simulink model "wheel_leg"  (R2024b)
settings: Solver=FixedStepAuto  StartTime=0.0  StopTime=10  FixedStep=0.001  RelTol=1e-3  AbsTol=1e-3  EnableMultiTasking=on
model workspace: external: MATLAB File UseBodyVel.m (data not in the file)
values from neighbouring files (symbols this model uses):
  g = 9.81    [LQR_calc.m]    (also in UseBodyVel.m)
  joint_distance = 0.11    [LQR_calc.m]    (also in UseBodyVel.m)
  l = -0.014    [LQR_calc.m]    (also in UseBodyVel.m)
  l_active_leg = 0.14    [LQR_calc.m]    (also in UseBodyVel.m)
  l_slave_leg = 0.24    [LQR_calc.m]    (also in UseBodyVel.m)
  M = 12    [LQR_calc.m]    (also in UseBodyVel.m)
  m_active_leg = 0.174    [LQR_calc.m]    (also in UseBodyVel.m)
  m_slave_leg = 0.180    (= 0.18)    [LQR_calc.m]    (also in UseBodyVel.m)
  mw = 0.58    [LQR_calc.m]    (also in UseBodyVel.m)
  N = mp*(x_ddot+L*theta_ddot*cos(theta)-L*theta_dot^2*sin(theta))+N_M    [UseBodyVel.m]
  X = [theta,theta_dot,x,x_dot,phi,phi_dot].'    [UseBodyVel.m]
undefined symbols (not defined in the file or in its folder): Y, Z
libraries: sm_lib x65, nesl_utility x25, dspfdesign x3
(part 1 of 3)
settings Model: Creator=kai  LastModifiedBy=kai
settings SolverCC: AutoScaleAbsTol=off  AlgebraicLoopSolver=TrustRegion  MaxZcPerStep=1
settings DataIOCC: LimitDataPoints=on  MaxDataPoints=10000
settings OptimizationCC: ReuseModelBlockBuffer=off  LifeSpan=inf
settings DebuggingCC: UnconnectedInputMsg=warning  UnconnectedOutputMsg=warning  UnconnectedLineMsg=warning  AllowSymbolicDim=off  SFUnexpectedBacktrackingDiag=warning  SFNoUnconditionalDefaultTransitionDiag=warning  SFExecutionAtInitializationDiag=none  ArithmeticOperatorsInVariantConditions=warning
settings ModelReferenceCC: EnableRefExpFcnMdlSchedulingChecks=on
settings SFSimCC: SimUseLocalCustomCode=off  CustomCodeUndefinedFunction=UseInterfaceOnly
settings RTWCC: RTWUseLocalCustomCode=off  GPUComputeCapability=3.5  DLArmComputeVersion=19.05
settings CodeAppCC: StateflowObjectComments=on
settings GRTTargetCC: TargetLangStandard=C89/C90 (ANSI)
settings ConfigComp: CovMetricSettings=dw  CovSaveCumulativeToWorkspaceVar=on  CovSaveSingleToWorkspaceVar=on  CovExternalEMLEnable=off  CovSFcnEnable=off
settings SimscapeCC: SimscapeLogType=all  SimscapeLogSimulationStatistics=on  SimscapeLogDataHistory=10000

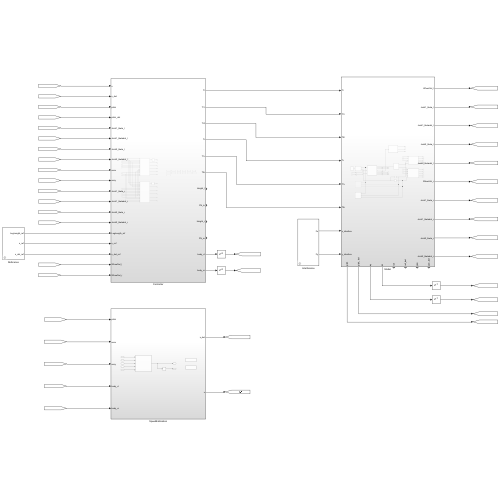
[thumbnail: Simulink's stored preview of the top-level diagram]
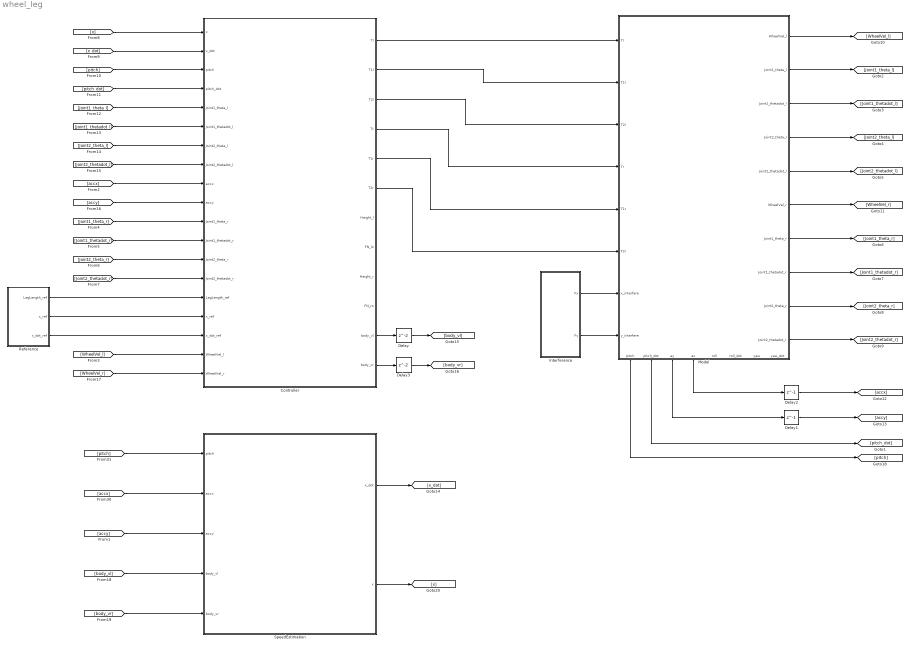
== system wheel_leg ==
  Controller : Subsystem
  Delay : Delay
  Delay1 : Delay  DelayLength=1
  Delay2 : Delay  DelayLength=1
  Delay3 : Delay
  Interference : Subsystem  mask{Fx=0, Fy=0}
      mask prompts: Fx "Fx（N）"; Fy "Fy（N）"
      mask DialogControl ParameterGroupVar Prompt: 参数
  Model : Subsystem
      settings: PortSchema="{\"entries\":[{\"content\":{\"sides\":[{\"content\":{\"connectorIds\":[\"In1\",\"In2\",\"In3\",\"In4\",\"In5\",\"In6\",\"In7\",\"In8\"]},\"type\":\"ConnectorPlacement.EquallySpacedRectSide\",\"uuid\":\"a2ef8d1c-db40-41d8-a076-97a3cc9cbcfc\"},{\"content\":{\"connectorIds\":[\"Out1\",\"Out2\",\"Out3\",\"Out4\",\"Out5\",\"Out6\",\"Out7\",\"Out8\",\"Out9\",\"Out10\"],\"side\":\"RIGHT\"},\"type\":\"ConnectorPlacement.EquallySpacedRectSide\",\"uuid\":\"78dabc19-8860-4beb-a8ed-91b17f10298d\"},{\"content\":{\"side\":\"TOP\"},\"type\":\"ConnectorPlacement.EquallySpacedRectSide\",\"uuid\":\"c54bf74f-6f46-45cf-a87a-01175e203e11\"},{\"content\":{\"connectorIds\":[\"Out11\",\"Out12\",\"Out13\",\"Out14\",\"Out15\",\"Out16\",\"Out17\",\"Out18\"],\"side\":\"BOTTOM\"},\"type\":\"ConnectorPlacement.EquallySpacedRectSide\",\"uuid\":\"b0255ca1-76d0-4c58-9ab3-44ef179b6807\"}]},\"type\":\"ConnectorPlacement.EquallySpacedConnector\",\"uuid\":\"6cb8f578-1c5f-4fff-8912-748653416d88\"}],\"packageUris\":[\"http://schema.mathworks.com/mf0/Connector/R2020b\"],\"version\":\"1.0\"}"
  Reference : Subsystem  mask{LegLength_expe=0.3, vel_expe=3, conti_time=7}
      mask prompts: LegLength_expe "腿长期望(m)"; vel_expe "速度期望(m/s)"; conti_time "速度持续时间(s)"
      mask DialogControl ParameterGroupVar Prompt: 参数
  SpeedEstimation : Subsystem
  wires:
  Model/2(Joint1_theta_l) -> [Joint1_theta_l]
  Model/3(Joint1_thetadot_l) -> [Joint1_thetadot_l]
  Model/4(Joint2_theta_l) -> [Joint2_theta_l]
  Model/5(Joint2_thetadot_l) -> [Joint2_thetadot_l]
  Model/7(Joint1_theta_r) -> [Joint1_theta_r]
  Model/8(Joint1_thetadot_r) -> [Joint1_thetadot_r]
  Model/9(Joint2_theta_r) -> [Joint2_theta_r]
  Model/10(Joint2_thetadot_r) -> [Joint2_thetadot_r]
  Model/1(WheelVel_l) -> [WheelVel_l]
  Model/6(WheelVel_r) -> [WheelVel_r]
  Model/11(pitch) -> [pitch]
  Model/12(pitch_dot) -> [pitch_dot]
  Model/13(ay) -> Delay1/1
  Delay1/1 -> [accy]
  Model/14(ax) -> Delay2/1
  Delay2/1 -> [accx]
  [pitch] -> SpeedEstimation/1(pitch)
  [accx] -> SpeedEstimation/2(accx)
  [x] -> Controller/1(x)
  [x_dot] -> Controller/2(x_dot)
  [pitch] -> Controller/3(pitch)
  [pitch_dot] -> Controller/4(pitch_dot)
  [Joint1_theta_l] -> Controller/5(Joint1_theta_l)
  [Joint1_thetadot_l] -> Controller/6(Joint1_thetadot_l)
  [Joint2_theta_l] -> Controller/7(Joint2_theta_l)
  [Joint2_thetadot_l] -> Controller/8(Joint2_thetadot_l)
  [accy] -> Controller/10(accy)
  [Joint1_theta_r] -> Controller/11(Joint1_theta_r)
  [Joint1_thetadot_r] -> Controller/12(Joint1_thetadot_r)
  [Joint2_theta_r] -> Controller/13(Joint2_theta_r)
  [Joint2_thetadot_r] -> Controller/14(Joint2_thetadot_r)
  Reference/1(LegLength_ref) -> Controller/15(LegLength_ref)
  Reference/2(x_ref) -> Controller/16(x_ref)
  Reference/3(x_dot_ref) -> Controller/17(x_dot_ref)
  Controller/1(Tl) -> Model/1(Tl)
  Controller/2(T1l) -> Model/2(T1l)
  Controller/3(T2l) -> Model/3(T2l)
  Controller/4(Tr) -> Model/4(Tr)
  Controller/5(T1r) -> Model/5(T1r)
  Controller/6(T2r) -> Model/6(T2r)
  [accx] -> Controller/9(accx)
  [accy] -> SpeedEstimation/3(accy)
  SpeedEstimation/1(x_dot) -> [x_dot]
  SpeedEstimation/2(x) -> [x]
  [WheelVel_l] -> Controller/18(WheelVel_l)
  [WheelVel_r] -> Controller/19(WheelVel_r)
  [body_vl] -> SpeedEstimation/4(body_vl)
  [body_vr] -> SpeedEstimation/5(body_vr)
  Controller/11(body_vl) -> Delay/1
  Delay/1 -> [body_vl]
  Controller/12(body_vr) -> Delay3/1
  Delay3/1 -> [body_vr]
  Interference/2(Fy) -> Model/8(y_interfere)
  Interference/1(Fx) -> Model/7(x_interfere)

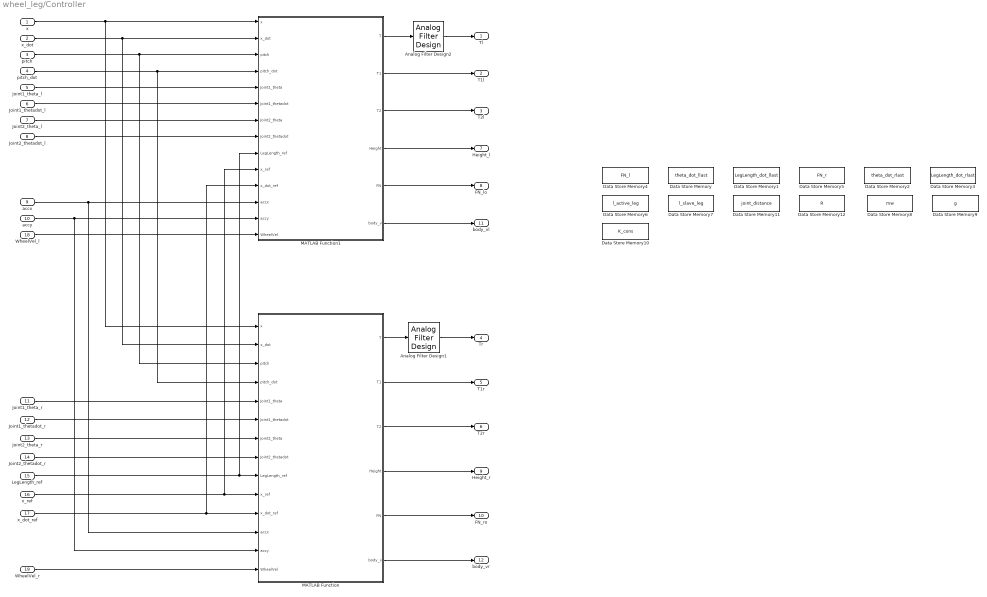
== system wheel_leg/Controller ==
  x : Inport
  x_dot : Inport  Port=2
  pitch : Inport  Port=3
  pitch_dot : Inport  Port=4
  Joint1_theta_l : Inport  Port=5
  Joint1_thetadot_l : Inport  Port=6
  Joint2_theta_l : Inport  Port=7
  Joint2_thetadot_l : Inport  Port=8
  accx : Inport  Port=9
  accy : Inport  Port=10
  Joint1_theta_r : Inport  Port=11
  Joint1_thetadot_r : Inport  Port=12
  Joint2_theta_r : Inport  Port=13
  Joint2_thetadot_r : Inport  Port=14
  LegLength_ref : Inport  Port=15
  x_ref : Inport  Port=16
  x_dot_ref : Inport  Port=17
  WheelVel_l : Inport  Port=18
  WheelVel_r : Inport  Port=19
  Analog Filter Design1 : dspfdesign/Analog Filter Design  method=Butterworth  filttype=Lowpass  N=1  Wlo=100  Whi=80  Rp=2  Rs=40
  Analog Filter Design2 : dspfdesign/Analog Filter Design  method=Butterworth  filttype=Lowpass  N=1  Wlo=100  Whi=80  Rp=2  Rs=40
  Data Store Memory : DataStoreMemory  DataStoreName=theta_dot_llast  WriteAfterWriteMsg=warning  ShowAdditionalParam=off  OutDataTypeStr=double
  Data Store Memory1 : DataStoreMemory  DataStoreName=LegLength_dot_llast  WriteAfterWriteMsg=warning  ShowAdditionalParam=off  OutDataTypeStr=double
  Data Store Memory10 : DataStoreMemory  DataStoreName=K_cons  WriteAfterWriteMsg=warning  InitialValue=K_cons  VectorParams1D=off  ShowAdditionalParam=off  OutDataTypeStr=double
  Data Store Memory11 : DataStoreMemory  DataStoreName=joint_distance  WriteAfterWriteMsg=warning  InitialValue=joint_distance  ShowAdditionalParam=off  OutDataTypeStr=double
  Data Store Memory12 : DataStoreMemory  DataStoreName=R  WriteAfterWriteMsg=warning  InitialValue=R  ShowAdditionalParam=off  OutDataTypeStr=double
  Data Store Memory2 : DataStoreMemory  DataStoreName=theta_dot_rlast  WriteAfterWriteMsg=warning  ShowAdditionalParam=off  OutDataTypeStr=double
  Data Store Memory3 : DataStoreMemory  DataStoreName=LegLength_dot_rlast  WriteAfterWriteMsg=warning  ShowAdditionalParam=off  OutDataTypeStr=double
  Data Store Memory4 : DataStoreMemory  DataStoreName=FN_l  WriteAfterWriteMsg=warning  InitialValue=70  ShowAdditionalParam=off  OutDataTypeStr=double
  Data Store Memory5 : DataStoreMemory  DataStoreName=FN_r  WriteAfterWriteMsg=warning  InitialValue=70  ShowAdditionalParam=off  OutDataTypeStr=double
  Data Store Memory6 : DataStoreMemory  DataStoreName=l_active_leg  WriteAfterWriteMsg=warning  InitialValue=l_active_leg  ShowAdditionalParam=off  OutDataTypeStr=double
  Data Store Memory7 : DataStoreMemory  DataStoreName=l_slave_leg  WriteAfterWriteMsg=warning  InitialValue=l_slave_leg  ShowAdditionalParam=off  OutDataTypeStr=double
  Data Store Memory8 : DataStoreMemory  DataStoreName=mw  WriteAfterWriteMsg=warning  InitialValue=mw  ShowAdditionalParam=off  OutDataTypeStr=double
  Data Store Memory9 : DataStoreMemory  DataStoreName=g  WriteAfterWriteMsg=warning  InitialValue=g  ShowAdditionalParam=off  OutDataTypeStr=double
  MATLAB Function : MATLAB Function  TreatAsAtomicUnit=on
  MATLAB Function1 : MATLAB Function  TreatAsAtomicUnit=on
  Tl : Outport
  T1l : Outport  Port=2
  T2l : Outport  Port=3
  Tr : Outport  Port=4
  T1r : Outport  Port=5
  T2r : Outport  Port=6
  Height_l : Outport  Port=7
  FN_lo : Outport  Port=8
  Height_r : Outport  Port=9
  FN_ro : Outport  Port=10
  body_vl : Outport  Port=11
  body_vr : Outport  Port=12
  wires:
  LegLength_ref/1 -> MATLAB Function/9(LegLength_ref), MATLAB Function1/9(LegLength_ref)
  MATLAB Function1/3(T2) -> T2l/1
  x_ref/1 -> MATLAB Function1/10(x_ref), MATLAB Function/10(x_ref)
  x_dot_ref/1 -> MATLAB Function1/11(x_dot_ref), MATLAB Function/11(x_dot_ref)
  MATLAB Function/1(T) -> Analog Filter Design1/1
  MATLAB Function/2(T1) -> T1r/1
  Analog Filter Design2/1 -> Tl/1
  MATLAB Function/3(T2) -> T2r/1
  Joint2_theta_r/1 -> MATLAB Function/7(Joint2_theta)
  Joint2_thetadot_r/1 -> MATLAB Function/8(Joint2_thetadot)
  MATLAB Function1/2(T1) -> T1l/1
  pitch_dot/1 -> MATLAB Function1/4(pitch_dot), MATLAB Function/4(pitch_dot)
  Joint1_thetadot_l/1 -> MATLAB Function1/6(Joint1_thetadot)
  Joint1_theta_r/1 -> MATLAB Function/5(Joint1_theta)
  MATLAB Function/5(FN) -> FN_ro/1
  x/1 -> MATLAB Function1/1(x), MATLAB Function/1(x)
  Joint1_thetadot_r/1 -> MATLAB Function/6(Joint1_thetadot)
  Joint2_theta_l/1 -> MATLAB Function1/7(Joint2_theta)
  Joint1_theta_l/1 -> MATLAB Function1/5(Joint1_theta)
  Analog Filter Design1/1 -> Tr/1
  accy/1 -> MATLAB Function/13(accy), MATLAB Function1/13(accy)
  Joint2_thetadot_l/1 -> MATLAB Function1/8(Joint2_thetadot)
  x_dot/1 -> MATLAB Function1/2(x_dot), MATLAB Function/2(x_dot)
  pitch/1 -> MATLAB Function1/3(pitch), MATLAB Function/3(pitch)
  MATLAB Function1/4(Height) -> Height_l/1
  MATLAB Function1/5(FN) -> FN_lo/1
  MATLAB Function/4(Height) -> Height_r/1
  accx/1 -> MATLAB Function/12(accx), MATLAB Function1/12(accx)
  MATLAB Function1/1(T) -> Analog Filter Design2/1
  WheelVel_l/1 -> MATLAB Function1/14(WheelVel)
  WheelVel_r/1 -> MATLAB Function/14(WheelVel)
  MATLAB Function1/6(body_v) -> body_vl/1
  MATLAB Function/6(body_v) -> body_vr/1

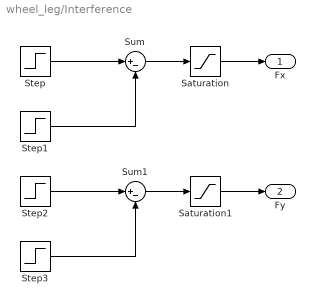
== system wheel_leg/Interference ==
  Saturation : Saturate  UpperLimit=80  LowerLimit=-80
  Saturation1 : Saturate  UpperLimit=100  LowerLimit=-100
  Step : Step  Time=0.5  After=Fx  SampleTime=0
  Step1 : Step  Time=0.6  After=Fx  SampleTime=0
  Step2 : Step  Time=0.5  After=Fy  SampleTime=0
  Step3 : Step  Time=0.6  After=Fy  SampleTime=0
  Sum : Sum  Inputs=|+-
  Sum1 : Sum  Inputs=|+-
  Fx : Outport
  Fy : Outport  Port=2
  wires:
  Step/1 -> Sum/1
  Step1/1 -> Sum/2
  Sum/1 -> Saturation/1
  Sum1/1 -> Saturation1/1
  Step3/1 -> Sum1/2
  Step2/1 -> Sum1/1
  Saturation/1 -> Fx/1
  Saturation1/1 -> Fy/1

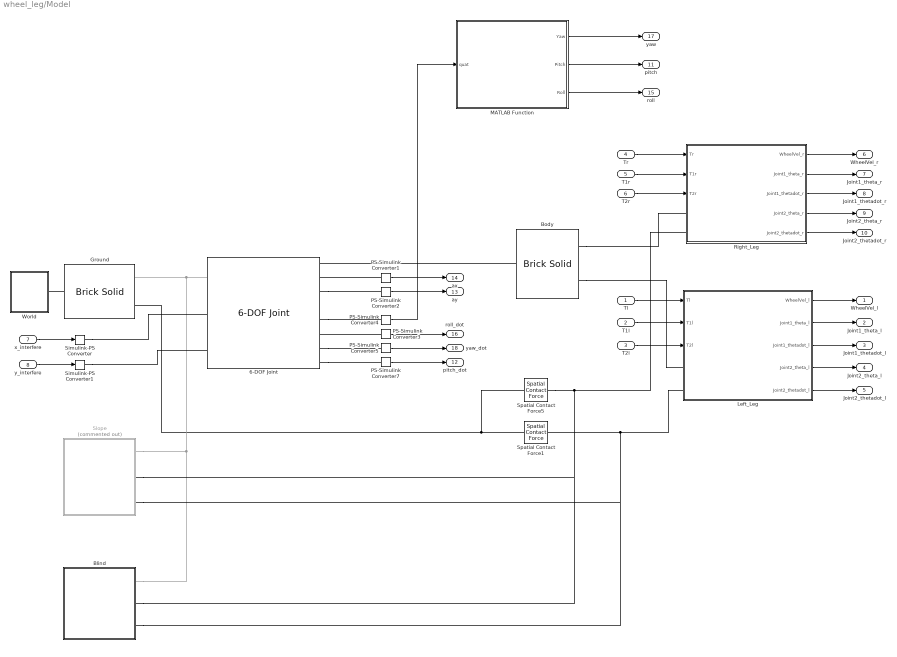
== system wheel_leg/Model ==
  Tl : Inport
  T1l : Inport  Port=2
  T2l : Inport  Port=3
  Tr : Inport  Port=4
  T1r : Inport  Port=5
  T2r : Inport  Port=6
  x_interfere : Inport  Port=7
  y_interfere : Inport  Port=8
  6-DOF Joint : sm_lib/Joints/6-DOF Joint  JointMode=Normal  CompositeWrenchDir=FollowerOnBase  CompositeWrenchFrame=BaseFrame  SenseConstraintForce=off  SenseConstraintTorque=off  SenseTotalForce=off  SenseTotalTorque=off  PxPositionTargetSpecify=off  PxPositionTargetPriority=High  PxPositionTargetValue=0  PxPositionTargetValueUnits=m  PxVelocityTargetSpecify=off  PxVelocityTargetPriority=High  PxVelocityTargetValue=0  PxVelocityTargetValueUnits=m/s  PxEquilibriumPosition=0  PxEquilibriumPositionUnits=m  PxSpringStiffness=0  PxSpringStiffnessUnits=N/m  PxDampingCoefficient=0  PxDampingCoefficientUnits=N/(m/s)  PxLowerLimitSpecify=off  PxLowerLimitBound=-1  PxLowerLimitBoundUnits=m  PxLowerLimitStiffness=1e6  PxLowerLimitStiffnessUnits=N/m  PxLowerLimitDamping=1e3  PxLowerLimitDampingUnits=N/(m/s)  PxLowerLimitTransitionRegionWidth=1e-4  PxLowerLimitTransitionRegionWidthUnits=m  PxUpperLimitSpecify=off  PxUpperLimitBound=1  PxUpperLimitBoundUnits=m  PxUpperLimitStiffness=1e6  PxUpperLimitStiffnessUnits=N/m  PxUpperLimitDamping=1e3  PxUpperLimitDampingUnits=N/(m/s)  PxUpperLimitTransitionRegionWidth=1e-4  PxUpperLimitTransitionRegionWidthUnits=m  PxTorqueActuationMode=InputTorque  PxMotionActuationMode=ComputedMotion  PxSensePosition=off  PxSenseVelocity=off  PxSenseAcceleration=on  PxSenseTorqueForce=off  PxSenseLowerLimitTorqueForce=off  PxSenseUpperLimitTorqueForce=off  PyPositionTargetSpecify=on  PyPositionTargetPriority=High  PyPositionTargetValue=0.33  PyPositionTargetValueUnits=m  PyVelocityTargetSpecify=off  PyVelocityTargetPriority=High  PyVelocityTargetValue=0  PyVelocityTargetValueUnits=m/s  PyEquilibriumPosition=0  PyEquilibriumPositionUnits=m  PySpringStiffness=0  PySpringStiffnessUnits=N/m  PyDampingCoefficient=0  PyDampingCoefficientUnits=N/(m/s)  PyLowerLimitSpecify=off  PyLowerLimitBound=-1  PyLowerLimitBoundUnits=m  PyLowerLimitStiffness=1e6  PyLowerLimitStiffnessUnits=N/m  PyLowerLimitDamping=1e3  PyLowerLimitDampingUnits=N/(m/s)  PyLowerLimitTransitionRegionWidth=1e-4  PyLowerLimitTransitionRegionWidthUnits=m  PyUpperLimitSpecify=off  PyUpperLimitBound=1  PyUpperLimitBoundUnits=m  PyUpperLimitStiffness=1e6  PyUpperLimitStiffnessUnits=N/m  PyUpperLimitDamping=1e3  PyUpperLimitDampingUnits=N/(m/s)  PyUpperLimitTransitionRegionWidth=1e-4  PyUpperLimitTransitionRegionWidthUnits=m  PyTorqueActuationMode=InputTorque  PyMotionActuationMode=ComputedMotion  PySensePosition=off  PySenseVelocity=off  PySenseAcceleration=on  PySenseTorqueForce=off  PySenseLowerLimitTorqueForce=off  PySenseUpperLimitTorqueForce=off  PzPositionTargetSpecify=off  PzPositionTargetPriority=High  PzPositionTargetValue=0  PzPositionTargetValueUnits=m  PzVelocityTargetSpecify=off  PzVelocityTargetPriority=High  PzVelocityTargetValue=0  PzVelocityTargetValueUnits=m/s  PzEquilibriumPosition=0  PzEquilibriumPositionUnits=m  PzSpringStiffness=0  PzSpringStiffnessUnits=N/m  PzDampingCoefficient=0  PzDampingCoefficientUnits=N/(m/s)  PzLowerLimitSpecify=off  PzLowerLimitBound=-1  PzLowerLimitBoundUnits=m  PzLowerLimitStiffness=1e6  PzLowerLimitStiffnessUnits=N/m  PzLowerLimitDamping=1e3  PzLowerLimitDampingUnits=N/(m/s)  PzLowerLimitTransitionRegionWidth=1e-4  PzLowerLimitTransitionRegionWidthUnits=m  PzUpperLimitSpecify=off  PzUpperLimitBound=1  PzUpperLimitBoundUnits=m  PzUpperLimitStiffness=1e6  PzUpperLimitStiffnessUnits=N/m  PzUpperLimitDamping=1e3  PzUpperLimitDampingUnits=N/(m/s)  PzUpperLimitTransitionRegionWidth=1e-4  PzUpperLimitTransitionRegionWidthUnits=m  PzTorqueActuationMode=NoTorque  PzMotionActuationMode=ComputedMotion  PzSensePosition=off  PzSenseVelocity=off  PzSenseAcceleration=on  PzSenseTorqueForce=off  PzSenseLowerLimitTorqueForce=off  PzSenseUpperLimitTorqueForce=off  SphPositionTargetSpecify=off  SphPositionTargetPriority=High  SphPositionTargetRotationMethod=None  SphPositionTargetFollAlignAxisA=+X  SphPositionTargetBaseAlignAxisA=+Y  SphPositionTargetFollAlignAxisB=+Y  SphPositionTargetBaseAlignAxisB=+Z  SphPositionTargetRotationStandardAxis=+Z  SphPositionTargetRotationAngle=0.0  SphPositionTargetRotationAngleUnits=deg  SphPositionTargetRotationArbitraryAxis=[0 0 1]  SphPositionTargetRotationSequenceAxes=FollowerAxes  SphPositionTargetRotationSequence=XYX  SphPositionTargetRotationSequenceAngles=[0 0 0]  SphPositionTargetRotationSequenceAnglesUnits=deg  SphPositionTargetRotationMatrix=[1 0 0; 0 1 0; 0 0 1]  SphPositionTargetQuaternion=[1 0 0 0]  SphVelocityTargetSpecify=off  SphVelocityTargetPriority=High  SphVelocityTargetValue=[0 0 0]  SphVelocityTargetValueUnits=deg/s  SphVelocityTargetInFollowerFrame=on  SphEqPosRotationMethod=None  SphEqPosFollAlignAxisA=+X  SphEqPosBaseAlignAxisA=+Y  SphEqPosFollAlignAxisB=+Y  SphEqPosBaseAlignAxisB=+Z  SphEqPosRotationStandardAxis=+Z  SphEqPosRotationAngle=0.0  SphEqPosRotationAngleUnits=deg  SphEqPosRotationArbitraryAxis=[0 0 1]  SphEqPosRotationSequenceAxes=FollowerAxes  SphEqPosRotationSequence=XYX  SphEqPosRotationSequenceAngles=[0 0 0]  SphEqPosRotationSequenceAnglesUnits=deg  SphEqPosRotationMatrix=[1 0 0; 0 1 0; 0 0 1]  SphEqPosQuaternion=[1 0 0 0]  SphSpringStiffness=0  SphSpringStiffnessUnits=N*m/deg  SphDampingCoefficient=0  SphDampingCoefficientUnits=N*m/(deg/s)  SphLowerLimitSpecify=off  SphLowerLimitBound=15  SphLowerLimitBoundUnits=deg  SphLowerLimitStiffness=1e4  SphLowerLimitStiffnessUnits=N*m/deg  SphLowerLimitDamping=10  SphLowerLimitDampingUnits=N*m/(deg/s)  SphLowerLimitTransitionRegionWidth=0.1  SphLowerLimitTransitionRegionWidthUnits=deg  SphUpperLimitSpecify=off  SphUpperLimitBound=45  SphUpperLimitBoundUnits=deg  SphUpperLimitStiffness=1e4  SphUpperLimitStiffnessUnits=N*m/deg  SphUpperLimitDamping=10  SphUpperLimitDampingUnits=N*m/(deg/s)  SphUpperLimitTransitionRegionWidth=0.1  SphUpperLimitTransitionRegionWidthUnits=deg  SphTorqueActuationMode=NoTorque  SphActuateTorqueX=off  SphActuateTorqueY=off  SphActuateTorqueZ=off  SphActuateTorque=off  SphActuationFrame=BaseFrame  SphSensePosition=on  SphSenseVelocityX=on  SphSenseVelocityY=on  SphSenseVelocityZ=on  SphSenseVelocity=off  SphSenseAccelerationX=off  SphSenseAccelerationY=off  SphSenseAccelerationZ=off  SphSenseAcceleration=off  SphSenseLowerLimitTorqueMag=off  SphSenseUpperLimitTorqueMag=off  SphSensingFrame=BaseFrame
  Blind : Subsystem
  Body : sm_lib/Body Elements/Brick Solid  BrickDimensions=[0.2 0.1 0.3]  BrickDimensionsUnits=m  ExportEntireGeometry=off  InertiaType=CalculateFromGeometry  BasedOnType=Mass  Density=1000  DensityUnits=kg/m^3  Mass=M  MassUnits=kg  CenterOfMass=[0 0 0]  CenterOfMassUnits=m  MomentsOfInertia=[1 1 1]  MomentsOfInertiaUnits=kg*m^2  ProductsOfInertia=[0 0 0]  ProductsOfInertiaUnits=kg*m^2  GraphicType=FromGeometry  MarkerShape=Sphere  MarkerSize=10  GraphicVisPropType=SimpleVisualProperties  GraphicDiffuseColor=[1.0 1.0 0.2]  GraphicOpacity=1.0  GraphicSpecularColor=[0.5 0.5 0.5 1.0]  GraphicAmbientColor=[0.15 0.15 0.15 1.0]  GraphicEmissiveColor=[0.0 0.0 0.0 1.0]  GraphicShininess=75  DoExposeReferenceFrame=on  SerializedFrames=<Frames><Frame><Id>Frame1</Id><Value><Name>Right</Name><Origin><Source>GeometricFeature</Source><FeatureName>+z surface</FeatureName></Origin><PrimaryAxis><DefinedDirection>+Z</DefinedDirection><Source>ReferenceFrame</Source><SourceDirection>+Z</SourceDirection><FeatureName></FeatureName></PrimaryAxis><SecondaryAxis><DefinedDirection>+X</DefinedDirection><Source>ReferenceFrame</Source><SourceDirection>+X</SourceDirection><FeatureName></FeatureName></SecondaryAxis></Value></Frame><Frame><Id>Frame2</Id><Value><Name>Left</Name><Origin><Source>GeometricFeature</Source><FeatureName>-z surface</FeatureName></Origin><PrimaryAxis><DefinedDirection>+Z</DefinedDirection><Source>ReferenceFrame</Source><SourceDirection>+Z</SourceDirection><FeatureName></FeatureName></PrimaryAxis><SecondaryAxis><DefinedDirection>+X</DefinedDirection><Source>ReferenceFrame</Source><SourceDirection>+X</SourceDirection><FeatureName></FeatureName></SecondaryAxis></Value></Frame></Frames>
  Ground : sm_lib/Body Elements/Brick Solid  BrickDimensions=[100 0.01 10]  BrickDimensionsUnits=m  ExportEntireGeometry=on  InertiaType=CalculateFromGeometry  BasedOnType=Density  Density=1000  DensityUnits=kg/m^3  Mass=1  MassUnits=kg  CenterOfMass=[0 0 0]  CenterOfMassUnits=m  MomentsOfInertia=[1 1 1]  MomentsOfInertiaUnits=kg*m^2  ProductsOfInertia=[0 0 0]  ProductsOfInertiaUnits=kg*m^2  GraphicType=FromGeometry  MarkerShape=Sphere  MarkerSize=10  GraphicVisPropType=SimpleVisualProperties  GraphicDiffuseColor=[0 0 1]  GraphicOpacity=1.0  GraphicSpecularColor=[0.5 0.5 0.5 1.0]  GraphicAmbientColor=[0.15 0.15 0.15 1.0]  GraphicEmissiveColor=[0.0 0.0 0.0 1.0]  GraphicShininess=75  DoExposeReferenceFrame=on  SerializedFrames=<Frames><Frame><Id>Frame1</Id><Value><Name>Surface</Name><Origin><Source>GeometricFeature</Source><FeatureName>+y surface</FeatureName></Origin><PrimaryAxis><DefinedDirection>+Z</DefinedDirection><Source>ReferenceFrame</Source><SourceDirection>+Z</SourceDirection><FeatureName></FeatureName></PrimaryAxis><SecondaryAxis><DefinedDirection>+X</DefinedDirection><Source>ReferenceFrame</Source><SourceDirection>+X</SourceDirection><FeatureName></FeatureName></SecondaryAxis></Value></Frame></Frames>
  Left_Leg : Subsystem
  MATLAB Function : MATLAB Function  TreatAsAtomicUnit=on
  PS-Simulink Converter{1..5,7} (6 alike) : nesl_utility/PS-Simulink Converter  PhysicalDomain=network_engine_domain  SubClassName=ps_output  LeftPortType=input  RightPortType=output  PseudoPeriodic=off  Frequencies=[]  VectorFormat=inherit  Unit=inherit  AffineConversion=off
  Right_Leg : Subsystem
  Simulink-PS Converter : nesl_utility/Simulink-PS Converter  PhysicalDomain=network_engine_domain  SubClassName=ps_input  LeftPortType=input  RightPortType=output  PseudoPeriodic=off  Frequencies=[]  NoiseDistribution=none  NoiseParameters=[]  Unit=1  AffineConversion=off  FilteringAndDerivatives=provide  SimscapeFilterOrder=1  InputFilterTimeConstant=0.001  UdotUserProvided=0
  Simulink-PS Converter1 : nesl_utility/Simulink-PS Converter  PhysicalDomain=network_engine_domain  SubClassName=ps_input  LeftPortType=input  RightPortType=output  PseudoPeriodic=off  Frequencies=[]  NoiseDistribution=none  NoiseParameters=[]  Unit=1  AffineConversion=off  FilteringAndDerivatives=provide  SimscapeFilterOrder=1  InputFilterTimeConstant=0.001  UdotUserProvided=0
  Slope : Subsystem  Commented=on  mask{gradient=15, length=1.2}
      mask prompts: gradient "坡度(deg)"; length "坡长(m)"
      mask DialogControl ParameterGroupVar Prompt: 参数
  Spatial Contact Force1 : sm_lib/Forces and Torques/Spatial Contact Force  NormalForceType=SmoothSpringDamper  NormalStiffness=1e6  NormalStiffnessUnits=N/m  NormalDamping=1e3  NormalDampingUnits=N/(m/s)  NormalTransitionRegionWidth=1e-4  NormalTransitionRegionWidthUnits=m  FrictionType=SmoothStickSlip  CoefficientOfStaticFriction=0.5  CoefficientOfDynamicFriction=0.3  FrictionalCriticalVelocity=1e-3  FrictionalCriticalVelocityUnits=m/s  SenseContactSignal=off  SensePenetrationDepth=off  SenseSeparationDistance=off  SenseNormalForceMagnitude=off  SenseFrictionalForceMagnitude=off  SenseNormalVelocity=off  SenseTangentialVelocity=off  SenseContactBaseRotation=off  SenseContactBaseTranslation=off  SenseContactFollowerRotation=off  SenseContactFollowerTranslation=off  ZeroCrossDetectContactStartAndEnd=off
  Spatial Contact Force5 : sm_lib/Forces and Torques/Spatial Contact Force  NormalForceType=SmoothSpringDamper  NormalStiffness=1e6  NormalStiffnessUnits=N/m  NormalDamping=1e3  NormalDampingUnits=N/(m/s)  NormalTransitionRegionWidth=1e-4  NormalTransitionRegionWidthUnits=m  FrictionType=SmoothStickSlip  CoefficientOfStaticFriction=0.5  CoefficientOfDynamicFriction=0.3  FrictionalCriticalVelocity=1e-3  FrictionalCriticalVelocityUnits=m/s  SenseContactSignal=off  SensePenetrationDepth=off  SenseSeparationDistance=off  SenseNormalForceMagnitude=off  SenseFrictionalForceMagnitude=off  SenseNormalVelocity=off  SenseTangentialVelocity=off  SenseContactBaseRotation=off  SenseContactBaseTranslation=off  SenseContactFollowerRotation=off  SenseContactFollowerTranslation=off  ZeroCrossDetectContactStartAndEnd=off
  World : Subsystem
  WheelVel_l : Outport
  Joint1_theta_l : Outport  Port=2
  Joint1_thetadot_l : Outport  Port=3
  Joint2_theta_l : Outport  Port=4
  Joint2_thetadot_l : Outport  Port=5
  WheelVel_r : Outport  Port=6
  Joint1_theta_r : Outport  Port=7
  Joint1_thetadot_r : Outport  Port=8
  Joint2_theta_r : Outport  Port=9
  Joint2_thetadot_r : Outport  Port=10
  pitch : Outport  Port=11
  pitch_dot : Outport  Port=12
  ay : Outport  Port=13
  ax : Outport  Port=14
  roll : Outport  Port=15
  roll_dot : Outport  Port=16
  yaw : Outport  Port=17
  yaw_dot : Outport  Port=18
  wires:
  Tr/1 -> Right_Leg/1(Tr)
  T1r/1 -> Right_Leg/2(T1r)
  T2r/1 -> Right_Leg/3(T2r)
  Right_Leg/1(WheelVel_r) -> WheelVel_r/1
  Right_Leg/2(Joint1_theta_r) -> Joint1_theta_r/1
  Right_Leg/3(Joint1_thetadot_r) -> Joint1_thetadot_r/1
  Right_Leg/4(Joint2_theta_r) -> Joint2_theta_r/1
  Right_Leg/5(Joint2_thetadot_r) -> Joint2_thetadot_r/1
  Tl/1 -> Left_Leg/1(Tl)
  T1l/1 -> Left_Leg/2(T1l)
  T2l/1 -> Left_Leg/3(T2l)
  Left_Leg/1(WheelVel_l) -> WheelVel_l/1
  Left_Leg/2(Joint1_theta_l) -> Joint1_theta_l/1
  Left_Leg/3(Joint1_thetadot_l) -> Joint1_thetadot_l/1
  Left_Leg/4(Joint2_theta_l) -> Joint2_theta_l/1
  Left_Leg/5(Joint2_thetadot_l) -> Joint2_thetadot_l/1
  PS-Simulink Converter2/1 -> ay/1
  PS-Simulink Converter4/1 -> MATLAB Function/1(quat)
  PS-Simulink Converter7/1 -> pitch_dot/1
  MATLAB Function/2(Pitch) -> pitch/1
  PS-Simulink Converter1/1 -> ax/1
  MATLAB Function/3(Roll) -> roll/1
  PS-Simulink Converter3/1 -> roll_dot/1
  MATLAB Function/1(Yaw) -> yaw/1
  PS-Simulink Converter5/1 -> yaw_dot/1
  x_interfere/1 -> Simulink-PS Converter/1
  y_interfere/1 -> Simulink-PS Converter1/1
  connections:
  Spatial Contact Force1/LConn1 -- Spatial Contact Force5/LConn1 -- Ground/LConn2
  Slope/LConn1 -- Ground/LConn1 -- 6-DOF Joint/LConn1 -- Blind/LConn1
  Body/RConn1 -- 6-DOF Joint/RConn1
  Ground/RConn1 -- World/RConn1
  Body/LConn1 -- Right_Leg/LConn1
  Left_Leg/LConn2 -- Blind/LConn3 -- Slope/LConn3 -- Spatial Contact Force1/RConn1
  Body/LConn2 -- Left_Leg/LConn1
  6-DOF Joint/RConn3 -- PS-Simulink Converter2/LConn1
  6-DOF Joint/RConn5 -- PS-Simulink Converter4/LConn1
  6-DOF Joint/RConn8 -- PS-Simulink Converter7/LConn1
  PS-Simulink Converter1/LConn1 -- 6-DOF Joint/RConn2
  PS-Simulink Converter3/LConn1 -- 6-DOF Joint/RConn6
  6-DOF Joint/RConn7 -- PS-Simulink Converter5/LConn1
  Spatial Contact Force5/RConn1 -- Blind/LConn2 -- Slope/LConn2 -- Right_Leg/LConn2
  Simulink-PS Converter/RConn1 -- 6-DOF Joint/LConn2
  Simulink-PS Converter1/RConn1 -- 6-DOF Joint/LConn3

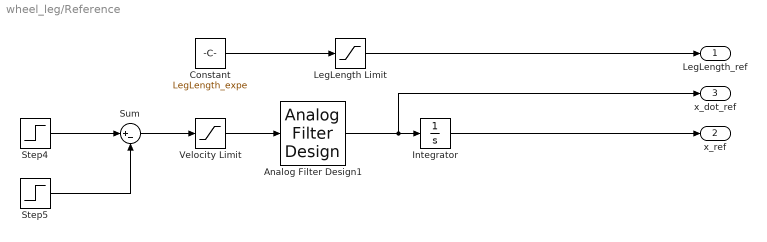
== system wheel_leg/Reference ==
  Analog Filter Design1 : dspfdesign/Analog Filter Design  method=Butterworth  filttype=Lowpass  N=1  Wlo=1  Whi=80  Rp=2  Rs=40
  Constant : Constant  Value=LegLength_expe
  Integrator : Integrator
  LegLength Limit : Saturate  UpperLimit=0.3  LowerLimit=0.1
  Step4 : Step  Time=0.3  After=vel_expe  SampleTime=0
  Step5 : Step  Time=0.3+conti_time  After=vel_expe  SampleTime=0
  Sum : Sum  Inputs=|+-
  Velocity Limit : Saturate  UpperLimit=3  LowerLimit=-3
  LegLength_ref : Outport
  x_ref : Outport  Port=2
  x_dot_ref : Outport  Port=3
  wires:
  Constant/1 -> LegLength Limit/1
  Integrator/1 -> x_ref/1
  LegLength Limit/1 -> LegLength_ref/1
  Step4/1 -> Sum/1
  Step5/1 -> Sum/2
  Sum/1 -> Velocity Limit/1
  Velocity Limit/1 -> Analog Filter Design1/1
  Analog Filter Design1/1 -> x_dot_ref/1, Integrator/1

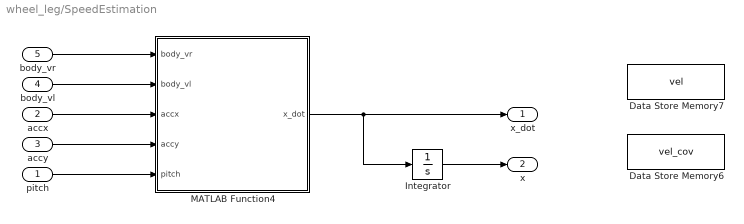
== system wheel_leg/SpeedEstimation ==
  pitch : Inport
  accx : Inport  Port=2
  accy : Inport  Port=3
  body_vl : Inport  Port=4
  body_vr : Inport  Port=5
  Data Store Memory6 : DataStoreMemory  DataStoreName=vel_cov  WriteAfterWriteMsg=warning  InitialValue=100  ShowAdditionalParam=off  OutDataTypeStr=double
  Data Store Memory7 : DataStoreMemory  DataStoreName=vel  WriteAfterWriteMsg=warning  ShowAdditionalParam=off  OutDataTypeStr=double
  Integrator : Integrator
  MATLAB Function4 : MATLAB Function  TreatAsAtomicUnit=on
  x_dot : Outport
  x : Outport  Port=2
  wires:
  MATLAB Function4/1(x_dot) -> x_dot/1, Integrator/1
  Integrator/1 -> x/1
  accx/1 -> MATLAB Function4/3(accx)
  pitch/1 -> MATLAB Function4/5(pitch)
  accy/1 -> MATLAB Function4/4(accy)
  body_vl/1 -> MATLAB Function4/2(body_vl)
  body_vr/1 -> MATLAB Function4/1(body_vr)

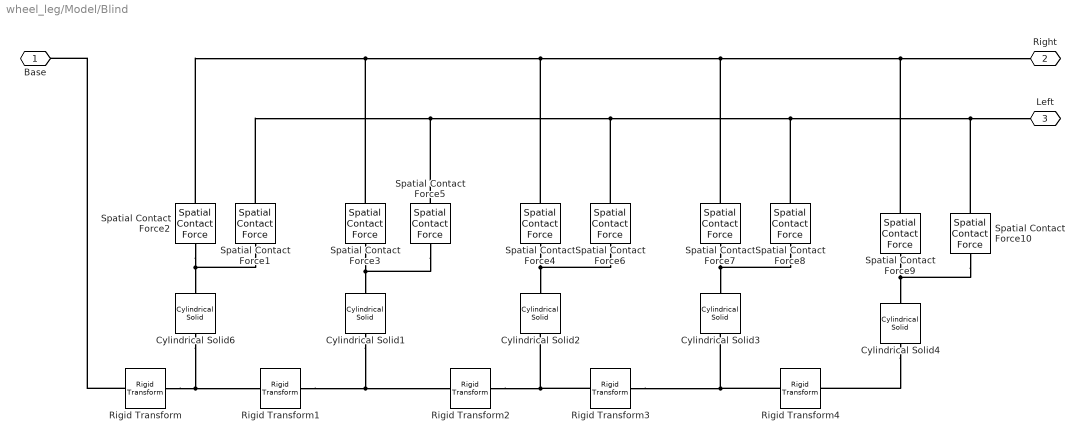
== system wheel_leg/Model/Blind ==
  Cylindrical Solid{1..4,6} (5 alike) : sm_lib/Body Elements/Cylindrical Solid  CylinderRadius=0.025  CylinderRadiusUnits=m  CylinderLength=10  CylinderLengthUnits=m  ExportEntireGeometry=on  InertiaType=CalculateFromGeometry  BasedOnType=Mass  Density=1000  DensityUnits=kg/m^3  Mass=0  MassUnits=kg  CenterOfMass=[0 0 0]  CenterOfMassUnits=m  MomentsOfInertia=[1 1 1]  MomentsOfInertiaUnits=kg*m^2  ProductsOfInertia=[0 0 0]  ProductsOfInertiaUnits=kg*m^2  GraphicType=FromGeometry  MarkerShape=Sphere  MarkerSize=10  GraphicVisPropType=SimpleVisualProperties  GraphicDiffuseColor=[1.0 0.6 0.6]  GraphicOpacity=1.0  GraphicSpecularColor=[0.5 0.5 0.5 1.0]  GraphicAmbientColor=[0.15 0.15 0.15 1.0]  GraphicEmissiveColor=[0.0 0.0 0.0 1.0]  GraphicShininess=75  DoExposeReferenceFrame=on  SerializedFrames=<Frames/>
  Rigid Transform : sm_lib/Frames and Transforms/Rigid Transform  RotationMethod=None  FollAlignAxisA=+X  BaseAlignAxisA=+Y  FollAlignAxisB=+Y  BaseAlignAxisB=+Z  RotationStandardAxis=+Z  RotationAngle=0.0  RotationAngleUnits=deg  RotationArbitraryAxis=[0 0 1]  RotationSequenceAxes=FollowerAxes  RotationSequence=XYX  RotationSequenceAngles=[0 0 0]  RotationSequenceAnglesUnits=deg  RotationMatrix=[1 0 0; 0 1 0; 0 0 1]  Quaternion=[1 0 0 0]  TranslationMethod=Cartesian  TranslationCartesianOffset=[10 -0.015 0]  TranslationCartesianOffsetUnits=m  TranslationStandardAxis=+Z  TranslationStandardOffset=0  TranslationStandardOffsetUnits=m  TranslationROffset=0  TranslationROffsetUnits=m  TranslationThetaOffset=0  TranslationThetaOffsetUnits=deg  TranslationZOffset=0  TranslationZOffsetUnits=m
  Rigid Transform{1..4} (4 alike) : sm_lib/Frames and Transforms/Rigid Transform  RotationMethod=None  FollAlignAxisA=+X  BaseAlignAxisA=+Y  FollAlignAxisB=+Y  BaseAlignAxisB=+Z  RotationStandardAxis=+Z  RotationAngle=0.0  RotationAngleUnits=deg  RotationArbitraryAxis=[0 0 1]  RotationSequenceAxes=FollowerAxes  RotationSequence=XYX  RotationSequenceAngles=[0 0 0]  RotationSequenceAnglesUnits=deg  RotationMatrix=[1 0 0; 0 1 0; 0 0 1]  Quaternion=[1 0 0 0]  TranslationMethod=Cartesian  TranslationCartesianOffset=[0.24 0 0]  TranslationCartesianOffsetUnits=m  TranslationStandardAxis=+Z  TranslationStandardOffset=0  TranslationStandardOffsetUnits=m  TranslationROffset=0  TranslationROffsetUnits=m  TranslationThetaOffset=0  TranslationThetaOffsetUnits=deg  TranslationZOffset=0  TranslationZOffsetUnits=m
  Spatial Contact Force{1..10} (10 alike) : sm_lib/Forces and Torques/Spatial Contact Force  NormalForceType=SmoothSpringDamper  NormalStiffness=1e6  NormalStiffnessUnits=N/m  NormalDamping=1e3  NormalDampingUnits=N/(m/s)  NormalTransitionRegionWidth=1e-4  NormalTransitionRegionWidthUnits=m  FrictionType=SmoothStickSlip  CoefficientOfStaticFriction=0.5  CoefficientOfDynamicFriction=0.3  FrictionalCriticalVelocity=1e-3  FrictionalCriticalVelocityUnits=m/s  SenseContactSignal=off  SensePenetrationDepth=off  SenseSeparationDistance=off  SenseNormalForceMagnitude=off  SenseFrictionalForceMagnitude=off  SenseNormalVelocity=off  SenseTangentialVelocity=off  SenseContactBaseRotation=off  SenseContactBaseTranslation=off  SenseContactFollowerRotation=off  SenseContactFollowerTranslation=off  ZeroCrossDetectContactStartAndEnd=off
  Base : PMIOPort  Side=Left
  Right : PMIOPort  Port=2  Side=Left
  Left : PMIOPort  Port=3  Side=Left
  connections:
  Rigid Transform/RConn1 -- Rigid Transform1/LConn1 -- Cylindrical Solid6/RConn1
  Spatial Contact Force3/LConn1 -- Spatial Contact Force5/LConn1 -- Cylindrical Solid1/LConn1
  Spatial Contact Force2/LConn1 -- Spatial Contact Force1/LConn1 -- Cylindrical Solid6/LConn1
  Rigid Transform1/RConn1 -- Cylindrical Solid1/RConn1 -- Rigid Transform2/LConn1
  Spatial Contact Force4/LConn1 -- Spatial Contact Force6/LConn1 -- Cylindrical Solid2/LConn1
  Rigid Transform2/RConn1 -- Rigid Transform3/LConn1 -- Cylindrical Solid2/RConn1
  Rigid Transform/LConn1 -- Base/RConn1
  Spatial Contact Force2/RConn1 -- Spatial Contact Force3/RConn1 -- Spatial Contact Force7/RConn1 -- Spatial Contact Force9/RConn1 -- Right/RConn1 -- Spatial Contact Force4/RConn1
  Spatial Contact Force1/RConn1 -- Spatial Contact Force5/RConn1 -- Spatial Contact Force6/RConn1 -- Spatial Contact Force8/RConn1 -- Spatial Contact Force10/RConn1 -- Left/RConn1
  Spatial Contact Force8/LConn1 -- Spatial Contact Force7/LConn1 -- Cylindrical Solid3/LConn1
  Rigid Transform3/RConn1 -- Rigid Transform4/LConn1 -- Cylindrical Solid3/RConn1
  Spatial Contact Force9/LConn1 -- Spatial Contact Force10/LConn1 -- Cylindrical Solid4/LConn1
  Cylindrical Solid4/RConn1 -- Rigid Transform4/RConn1
